simulink model "mymodel_sim"  (R2019b)
settings: Solver=ode45  StartTime=0.0  StopTime=20  RelTol=1e-3
values from neighbouring files (symbols this model uses):
  stepf = 10    [Exercises2.m]    (also in MassSpringDamperSys.m; RunMyModelSim.m)
  stepi = 2    [Exercises2.m]    (also in MassSpringDamperSys.m; RunMyModelSim.m = 0)
  stept = 1    [Exercises2.m]    (also in MassSpringDamperSys.m; RunMyModelSim.m)
  x0 = [0,0]    [Exercises2.m]    (also in MassSpringDamperSys.m; RunMyModelSim.m = 0)
settings Model: Creator=don  LastModifiedBy=don
settings DataIOCC: TimeSaveName=mytime

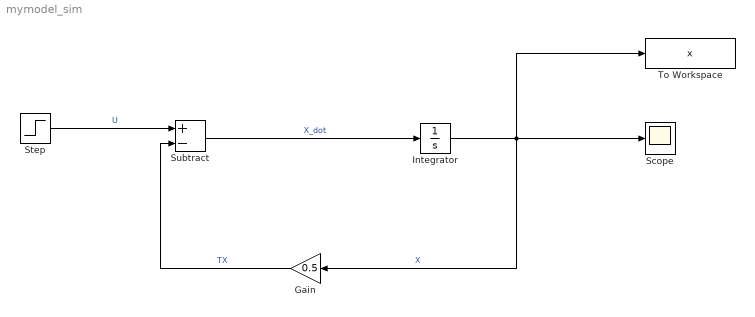
== system mymodel_sim ==
  Gain : Gain  Gain=0.5
  Integrator : Integrator  InitialCondition=x0
  Scope : Scope
  Step : Step  Time=stept  Before=stepi  After=stepf  SampleTime=0
  Subtract : Sum  Inputs=+-
  To Workspace : ToWorkspace  VariableName=x  SampleTime=-1
  wires:
  Step/1 -> Subtract/1  "U"
  Subtract/1 -> Integrator/1  "X_dot"
  Integrator/1 -> Gain/1, Scope/1, To Workspace/1  "X"
  Gain/1 -> Subtract/2  "TX"
